simulink model "rtlsdr_am_fdm_demod"  (R2014b)
settings: Solver=ode45  StartTime=0.0  StopTime=60  RelTol=1e-3
PreLoadFcn:
  | %%%%%%%%%%%%%%%%%%%%%%%%%%%%%%%%%%%%%%%%%%%%%%%%%%%%%%%%%%%%%%%%%%%%%%%%%%%
  | % check to see if Simulink library folder is missing from the MATLAB path %
  | %%%%%%%%%%%%%%%%%%%%%%%%%%%%%%%%%%%%%%%%%%%%%%%%%%%%%%%%%%%%%%%%%%%%%%%%%%%
  | if isempty(strfind(path, 'rtlsdr_book_library'))
  | 
  |     % create error window
  |     fig_error = figure(...
  |         'Name', 'Error: RTL-SDR Book Library',...
  |         'Toolbar','none',...
  |         'MenuBar','none',...
  |         'NumberTitle','off',...
  |         'Resize','off',...
  |         'WindowStyle','modal');
  |     fig_error.Position(3) = 600;
  |     fig_error.Position(4) = 150;
  |     fig_axes = axes(...
  |         'Parent',fig_error,...
  |         'Position',[0,0,1,1],...
  |         'visible','off');
  |     % error message
  |     t_title = text(.05,.8,...
  |         'MISSING DIRECTORIES',...
  |         'FontSize',11.5);
  |     t_body = text(.075,.6,...
  |         [{'Simulink cannot find the  \it{<root>}\rm / \it{rtlsdr\_book\_library}\rm  folder in the \it{MATLAB Path}\rm.'},...
  |         {'Please set the MATLAB path following the instructions given in Exercise 2.4.'}],...
  |         'FontSize',10.5);
  |     % buttons
  |     btn_path = uicontrol(...
  |         'Parent',fig_error,...
  |         'String','Set Path Now',...
  |         'FontSize',10,...
  |         'Callback', 'pathtool; close(fig_error);',...
  |         'Position', [fig_error.Position(3)/2-210, 30, 200, 30]);
  |     btn_abort = uicontrol(...
  |         'Parent',fig_error,...
  |         'String','No thanks',...
  |         'FontSize',10,...
  |         'Callback', 'close(fig_error); abort=1;',...
  |         'Position', [fig_error.Position(3)/2+10, 30, 200, 30]);
  | 
  |     % pause to allow user to interact with error box
  |     uiwait(fig_error);
  | 
  |     % abort simulation
  |     try
  |         if abort==1
  |             set_param(gcs, 'SimulationCommand', 'stop');
  |         end
  |     end
  | 
  |     % if user has set path, allow diagram to be updated
  |     if ~exist('abort','var')
  |         % create error window
  |         fig_update = figure(...
  |             'Name', 'Update Diagram',...
  |             'Toolbar','none',...
  |             'MenuBar','none',...
  |             'NumberTitle','off',...
  |             'Resize','off');
  |         fig_update.Position(3) = 400;
  |         fig_update.Position(4) = 120;
  |         fig_axes = axes(...
  |             'Parent',fig_update,...
  |             'Position',[0,0,1,1],...
  |             'visible','off');
  |         % instruction message
  |         t_body = text(.075,.7,...
  |             'Once you have set the path, update the block diagram',...
  |             'FontSize',10.5);
  |         % button
  |         btn_update = uicontrol(...
  |             'Parent',fig_update,...
  |             'String','Update Block Diagram',...
  |             'FontSize',10,...
  |             'Callback', 'set_param(gcs,''SimulationCommand'',''update''); close(gcf)',...
  |             'Position', [fig_update.Position(3)/2-100, 30, 200, 30]);
  |     end
  | 
  |     % clear error components
  |     clear('fig_error','fig_update','fig_axes','t_title','t_body','btn_path','btn_abort','btn_update','abort');
  | 
  | end
  | %%%%%%%%%%%%%%%%%%%%%%%%%%%%%%%%%%%%%%%%%%%%%%%%%%%%%%%%%%%%%%%%%%%%%%%%%%%
undefined symbols (not defined in the file or in its folder): dfilt, fdesignblkfcn, gcbh, startfcn_spectrum_analyzer, startfcn_time_scope
libraries: dsparch4 x4, rtlsdr_book_library x2, dspmlti4 x1, sdrrlib x1, dspsnks4 x1
CloseFcn:
  | closefcn_model;
Description:
  | Software, Simulation Examples and Design Exercises Licence Agreement
  | 
  | This license agreement refers to the simulation examples, design exercises and files,
  | and associated software MATLAB and Simulink resources that accompany the book:
  | 
  |      Title: Software Defined Radio using MATLAB & Simulink and the RTL-SDR
  |      Published by Strathclyde Academic Media, 2015
  |      Authored by Robert W. Stewart, Kenneth W. Barlee, Dale S.W. Atkinson,
  |      and Louise H. Crockett
  | 
  | and made available as a download from, www.desktopSDR.com or variously acquired
  | by other means such as via USB storage, cloud storage, disk or any other electronic
  | or optical or magnetic storage mechanism. These files and associated software may
  | be used subject to the terms of agreement of the conditions below:
  | 
  |     Copyright © 2015 Robert W. Stewart, Kenneth W. Barlee, Dale S.W. Atkinson,
  |     and Louise H. Crockett
  |     All rights reserved.
  | 
  | Redistribution and use in source and binary forms, with or without modification, are
  | permitted provided that the following conditions are met:
  | 
  |    1.  Redistributions of source code must retain the above copyright notice, this list of
  |         conditions and the following disclaimer.
  | 
  |    2.  Redistributions in binary form must reproduce the above copyright notice, this
  |         list of conditions and the following disclaimer in the documentation and/or other
  |         materials provided with the distribution.
  | 
  |    3.  Neither the name of the copyright holder nor the names of its contributors may
  |         be used to endorse or promote products derived from this software without
  |         specific prior written permission.
  | 
  |    4.  In all cases, the software is, and all modifications and derivatives of the
  |         software shall be, licensed to you solely for use in conjunction with The
  |         MathWorks, Inc. products and service offerings.
  | 
  | THIS SOFTWARE IS PROVIDED BY THE COPYRIGHT HOLDERS AND CONTRIBUTORS
  | "AS IS" AND ANY EXPRESS OR IMPLIED WARRANTIES, INCLUDING, BUT NOT LIMITED
  | TO, THE IMPLIED WARRANTIES OF MERCHANTABILITY AND FITNESS FOR A
  | PARTICULAR PURPOSE ARE DISCLAIMED. IN NO EVENT SHALL THE COPYRIGHT
  | HOLDER OR CONTRIBUTORS BE LIABLE FOR ANY DIRECT, INDIRECT, INCIDENTAL,
  | SPECIAL, EXEMPLARY, OR CONSEQUENTIAL DAMAGES (INCLUDING, BUT NOT
  | LIMITED TO, PROCUREMENT OF SUBSTITUTE GOODS OR SERVICES; LOSS OF USE,
  | DATA, OR PROFITS; OR BUSINESS INTERRUPTION) HOWEVER CAUSED AND ON ANY
  | THEORY OF LIABILITY, WHETHER IN CONTRACT, STRICT LIABILITY, OR TORT
  | (INCLUDING NEGLIGENCE OR OTHERWISE) ARISING IN ANY WAY OUT OF THE USE
  | OF THIS SOFTWARE, EVEN IF ADVISED OF THE POSSIBILITY OF SUCH DAMAGE.
  | 
  | 
  | Audio Tracks used in Simulations Examples and Design Exercises
  | 
  | The music and vocal files used within the Examples files and software within the book
  | were variously written, arranged, performed, recorded and produced by Garrey Rice,
  | Adam Struth, Jamie Struth, Iain Thistlethwaite and also Marshall Craigmyle who
  | collectively, and individually where appropriate, assert and retain all of their copyright,
  | performance and artistic rights. Permission to use and reproduce this music is
  | granted for all purposes associated with MATLAB and Simulink software and the
  | simulation examples and design exercises files that accompany this book. Requests to
  | use the music for any other purpose should be directed to: info@desktopSDR.com.
  | For information on music track names, full credits, and links to the musicians please
  | refer to www.desktopSDR.com/more/audio.
settings Model: Creator=desktopSDR Team  LastModifiedBy=desktopSDR Team
settings DataIOCC: LimitDataPoints=off  SaveOutput=off  SignalLogging=off  SaveTime=off

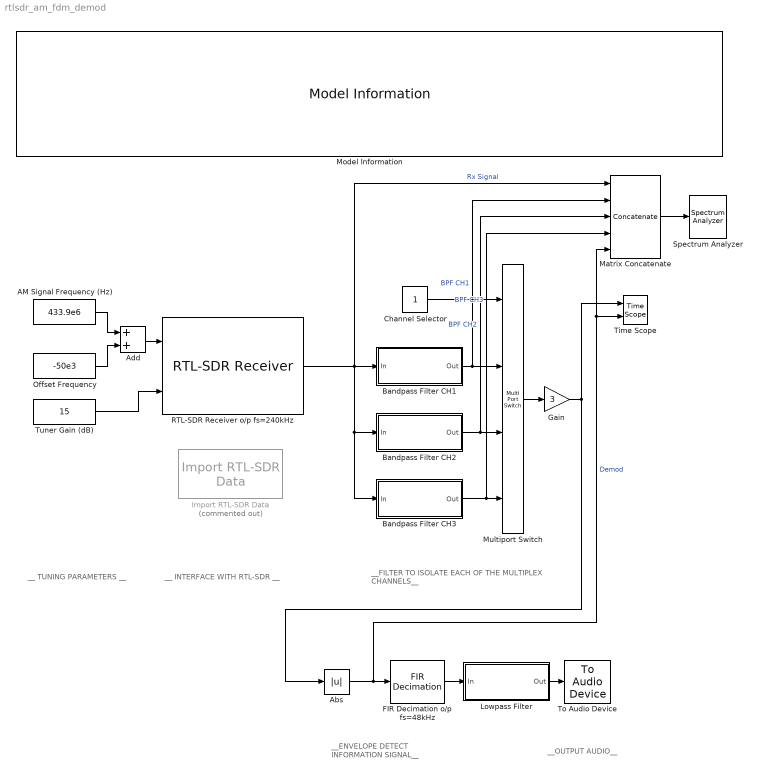
== system rtlsdr_am_fdm_demod ==
  note: __ TUNING PARAMETERS __
  note: __ INTERFACE WITH RTL-SDR __
  note: __FILTER TO ISOLATE EACH
      | OF THE MULTIPLEX CHANNELS__
  note: __OUTPUT AUDIO__
  note: __ENVELOPE DETECT
      | INFORMATION SIGNAL__
  AM Signal Frequency (Hz) : Constant  Value=433.9e6
  Abs : Abs
  Add : Sum
  Bandpass Filter CH1 : Subsystem  DialogController=fdesignblkfcn  InitFcn=fdesignblkfcn(gcbh, {'InitFcn'});  mask(Bandpass Filter){}
      mask help: Design a bandpass filter
      settings: CopyFcn=fdesignblkfcn(gcbh, {'CopyFcn'});
      mask Help: helpview(mapfilelocation('dsp'), 'dspbandpassfilter');
      mask Display: disp('Bandpass');
  Bandpass Filter CH2 : Subsystem  DialogController=fdesignblkfcn  InitFcn=fdesignblkfcn(gcbh, {'InitFcn'});  mask(Bandpass Filter){}
      mask help: Design a bandpass filter
      settings: CopyFcn=fdesignblkfcn(gcbh, {'CopyFcn'});
      mask Help: helpview(mapfilelocation('dsp'), 'dspbandpassfilter');
      mask Display: disp('Bandpass');
  Bandpass Filter CH3 : Subsystem  DialogController=fdesignblkfcn  InitFcn=fdesignblkfcn(gcbh, {'InitFcn'});  mask(Bandpass Filter){}
      mask help: Design a bandpass filter
      settings: CopyFcn=fdesignblkfcn(gcbh, {'CopyFcn'});
      mask Help: helpview(mapfilelocation('dsp'), 'dspbandpassfilter');
      mask Display: disp('Bandpass');
  Channel Selector : Constant
  FIR Decimation o/p fs=48kHz : dspmlti4/FIR Decimation  h=firpm(100, [0 15e3 20e3 (240e3/2)]/(240e3/2), [1 1 0 0], [1 1], 20)  D=5  filtStruct=Direct form  framing=Allow multirate processing  inputOffset=0  outputBufInitCond=0  InputProcessing=Columns as channels (frame based)  firstCoeffDataTypeStr=Inherit: Same word length as input  firstCoeffLastDataTypeStr=Inherit: Same word length as input  firstCoeffMin=[]  firstCoeffMax=[]  outputDataTypeStr=Inherit: Same as accumulator  outputLastDataTypeStr=Inherit: Same as accumulator  outputMin=[]  outputMax=[]  roundingMode=Floor  overflowMode=off  FilterSource=Specify via dialog  FilterObject=Hm_firdecim
      settings: allowOverrides=off
  Gain : Gain  Gain=3
  Import RTL-SDR Data : rtlsdr_book_library/Additional Tools/Import RTL-SDR Data  Commented=on  filename=rec_data/am_fdm.mat  frm_size=4096  data_type=single
  Lowpass Filter : Subsystem  DialogController=fdesignblkfcn  InitFcn=fdesignblkfcn(gcbh, {'InitFcn'});  mask(Lowpass Filter){}
      mask help: Design a lowpass filter
      settings: CopyFcn=fdesignblkfcn(gcbh, {'CopyFcn'});
      mask Help: helpview(mapfilelocation('dsp'), 'dsplowpassfilter');
      mask Display: disp('Lowpass')
  Matrix Concatenate : Concatenate  NumInputs=5  Mode=Multidimensional array  ConcatenateDimension=2
  Model Information : rtlsdr_book_library/Additional Tools/Model Information/Model Information
  Multiport Switch : MultiPortSwitch
  Offset Frequency : Constant  Value=-50e3
  RTL-SDR Receiver o/p fs=240kHz : sdrrlib/RTL-SDR Receiver  SourceLibraryInfo="This block requires <a href=\"http://www.mathworks.com/hardware-support/rtl-sdr.html\">Communications System Toolbox Support Package for RTL-SDR Radio</a>"  sobjType=sdrr.internal.SDRRTLReceiverSL  IPAddress=0  dataUDPPort=-1  ctrlUDPPort=-1  subDeviceList=nosubdev  sdrBlockType=SDRBlockTypeSLT.SDRRxBlock  requester=UNUSED_BY_SFCN  sdrExecutionMode=SDRExecutionModeSLT.ExecModeHW  LostSamplesOutputPort=off  OutputDataType=single  FrameLength=4096  EnableBurstMode=off  NumFramesInBurst=20  BypassUserLogic=off  DecimatorSelect=DDC decimator  SourceSelect=RF data  SineAmplitude=16000  EnableInternalClock=off  BypassIQBalance=off  CenterFrequency=433.9e6-100e3  IFBandwidth=40e6  ADCRateSource=Dialog  ADCRate=240e3  CenterFrequencySource=Input port  GainSource=Input port  IntermediateFrequency=0  Gain=40  DecimationFactorSource=Dialog  DecimationFactor=512  RFFrequencyIsTunable=logical(1)  SampleTime=(4096)/(240e3)  IFBandwidthSource=Dialog  SineFrequency=30000  BypassDCBlockingFilter=off  IntermediateFrequencySource=Dialog  IQBalanceCoefficients=64  SkipAllHardwareResetAndInitialization=off  EnableIQCalibrationTable=on  CacheIQCalibrationTable=off  EnableOffsetTuning=off  EnableRTLAGC=off  EnableTestMode=off  EnableTunerAGC=off  FrequencyCorrectionSource=Dialog  FrequencyCorrection=0  NumMLBuffers=128  NumUSBBuffers=16  LatencyOutputPort=off  RTLCrystalFrequency=28800000  TunerCrystalFrequency=28800000
  Spectrum Analyzer : SpectrumAnalyzer  StartFcn=startfcn_spectrum_analyzer;
  Time Scope : TimeScope  StartFcn=startfcn_time_scope;  DefaultConfigurationName=spbscopes.TimeScopeBlockCfg  NumInputPorts=2
  To Audio Device : dspsnks4/To Audio Device  deviceName=Default  inheritSampleRate=on  sampleRate=44100  deviceDatatype=Determine from input data type  autoBufferSize=on  bufferSize=4096  queueDuration=1.0  defaultOutputChannelMapping=on  outputChannelMapping=1  outputNumUnderrunSamples=off
  Tuner Gain (dB) : Constant  Value=15
  wires:
  AM Signal Frequency (Hz)/1 -> Add/1
  Offset Frequency/1 -> Add/2
  Matrix Concatenate/1 -> Spectrum Analyzer/1
  Add/1 -> RTL-SDR Receiver o/p fs=240kHz/1
  Tuner Gain (dB)/1 -> RTL-SDR Receiver o/p fs=240kHz/2
  Lowpass Filter/1(Out) -> To Audio Device/1
  Channel Selector/1 -> Multiport Switch/1
  Bandpass Filter CH3/1(Out) -> Matrix Concatenate/4, Multiport Switch/4  "BPF CH3"
  Bandpass Filter CH2/1(Out) -> Matrix Concatenate/3, Multiport Switch/3  "BPF CH2"
  FIR Decimation o/p fs=48kHz/1 -> Lowpass Filter/1(In)
  Bandpass Filter CH1/1(Out) -> Matrix Concatenate/2, Multiport Switch/2  "BPF CH1"
  Multiport Switch/1 -> Gain/1
  Abs/1 -> Time Scope/2, Matrix Concatenate/5, FIR Decimation o/p fs=48kHz/1  "Demod"
  Gain/1 -> Time Scope/1, Abs/1
  RTL-SDR Receiver o/p fs=240kHz/1 -> Bandpass Filter CH3/1(In), Bandpass Filter CH2/1(In), Bandpass Filter CH1/1(In), Matrix Concatenate/1  "Rx Signal"

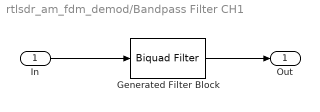
== system rtlsdr_am_fdm_demod/Bandpass Filter CH1 ==
  In : Inport
  Generated Filter Block : dsparch4/Biquad Filter  Tag=BlockMethodSubSystem  IIRFiltStruct=Direct form II  CoeffSource=Specify via dialog  BiQuadCoeffs=[0.48710578309185842 0.020274699864626225 0.47606726400774318 1 -0.3200568934772296 0.9510875417757314;0.61694390478008665 -0.57271773922302893 0.60189559689807448 1 -0.68371663134321814 0.94964854256260212;0.84000114524790004 0.45824504577674063 0.021305946041866301 1 -0.48832315180999453 0.90165549195060035;0.0064548478739541466 0.011389175960501097 0.0049921122031908582 1 -0.72821163596699334 0.034855521810121665;0.77833495194845737 -0.20151009399259803 0.77832234721342286 1 -0.28213942704351702 0.99443660184789129;2 -1.5345249628396347 1.9997202303570027 1 -0.74285445349198365 0.99437926899504725;0.68303493454046227 0.074580654630850063 0.062904140898226851 1 -0.38577358709267945 0.9184389811629543;0.038054397531435698 -0.029838005454256376 0.0052742626653348402 1 -0.60016342729911176 0.91586675515872462;0.81687912100239568 -0.19207817940590149 0.81368134800883141 1 -0.29088293607338106 0.97858989499573013;2 -1.5735978982408823 1.9913568136029411 1 -0.7264857258290689 0.97824331105542206]  a0Flag=Warning  IC=0  ICnum=0  ICden=0  InputProcessing=Columns as channels (frame based)  denAccumFracLength=30  denProdOutputFracLength=30  secondMemoryFracLength=15  roundingMode=Floor  overflowMode=off  ScaleValues=[0.048249460042969664;1;1;1;1;1;1;1;1;1;10.550556890003632]  optimizeScaleValues=off  ScaleValueMode=Specify via input port (g)  scaleValueFracLength=14  FilterSource=Specify via dialog  dfiltObjectName=dfilt.df2tsos([1 0.3 0.4],[1 0.1 0.2])
  Out : Outport
  wires:
  Generated Filter Block/1 -> Out/1
  In/1 -> Generated Filter Block/1

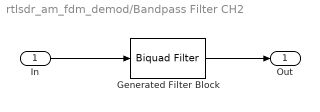
== system rtlsdr_am_fdm_demod/Bandpass Filter CH2 ==
  In : Inport
  Generated Filter Block : dsparch4/Biquad Filter  Tag=BlockMethodSubSystem  IIRFiltStruct=Direct form II  CoeffSource=Specify via dialog  BiQuadCoeffs=[0.67338527760443312 -0.26671696059651728 0.6083593445883243 1 -0.19930278069396612 0.95848462181243144;0.5841637340870659 0.29230149777999481 0.56667307615551432 1 0.19906120642328817 0.9582828801664226;0.149036042446199 0.016946608863773197 0.010962149262872629 1 -0.052041795111932465 0.90786508164551083;0.020481807136560625 0.0032274650327607547 0.00012161868746611722 1 0.051117066171290415 0.9077685137822048;0.88089444047624554 -0.23157465446878642 0.88081993658726632 1 -0.23868838376901563 0.99490529520038307;2 0.52571694552187798 1.9997830967396211 1 0.23871035705725224 0.9948917802055679;0.75363304099796768 -0.50601088924497151 0.63927957482421738 1 -0.14123666236621696 0.929598737259827;0.057396929567661487 0.037309121966942291 0.051540971083893876 1 0.14053864118672826 0.92931947808271609;0.89113560972214434 -0.25188520382892204 0.89037379535859118 1 -0.22797195313135205 0.98116025020292619;2 0.56543358427809076 1.9989110580547198 1 0.22796205762099908 0.98109487138402474]  a0Flag=Warning  IC=0  ICnum=0  ICden=0  InputProcessing=Columns as channels (frame based)  denAccumFracLength=30  denProdOutputFracLength=30  secondMemoryFracLength=15  roundingMode=Floor  overflowMode=off  ScaleValues=[0.041299783151138178;1;1;1;1;1;1;1;1;1;10.556598798294175]  optimizeScaleValues=off  ScaleValueMode=Specify via input port (g)  scaleValueFracLength=14  FilterSource=Specify via dialog  dfiltObjectName=dfilt.df2tsos([1 0.3 0.4],[1 0.1 0.2])
  Out : Outport
  wires:
  Generated Filter Block/1 -> Out/1
  In/1 -> Generated Filter Block/1

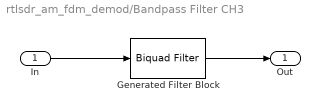
== system rtlsdr_am_fdm_demod/Bandpass Filter CH3 ==
  In : Inport
  Generated Filter Block : dsparch4/Biquad Filter  Tag=BlockMethodSubSystem  IIRFiltStruct=Direct form II  CoeffSource=Specify via dialog  BiQuadCoeffs=[0.60849794827942949 -0.39367779312989598 0.60510522232424568 1 -0.80225454616844827 0.94803791480656774;1.0827491135228735 -1.4017183159916566 1.0805570736721235 1 -1.1330291323642383 0.94553328874405862;-0.28844190743740877 -0.36640640350330222 -0.1161247491557328 1 -0.92719616379501202 0.87407382671627254;0.0051149879255016342 0.0084662498713601719 0.0035008355536301078 1 -0.41129230893568486 0.41217232074731847;0.87875947987193626 -0.67084490391661322 0.87832130941815556 1 -0.78328718222404869 0.99448369227738287;1.6407858750865425 -2 1.6404606425531527 1 -1.1968053935527578 0.99438971688497091;0.95363887304809736 -0.28707398288206454 0.11651775049576317 1 -0.8461554451210308 0.90205598979649637;0.026450365759947799 0.0097397859288686859 0.00089653680768698302 1 -1.0414658285428771 0.89903207911897964;0.76281842819729895 -0.56804251861329702 0.76239803937086215 1 -0.78624791416512241 0.97854881912371261;1.6201527105224738 -2 1.6195618818344955 1 -1.178676630833333 0.97790653821453]  a0Flag=Warning  IC=0  ICnum=0  ICden=0  InputProcessing=Columns as channels (frame based)  denAccumFracLength=30  denProdOutputFracLength=30  secondMemoryFracLength=15  roundingMode=Floor  overflowMode=off  ScaleValues=[0.04734822056392915;1;1;1;1;1;1;1;1;1;16.324610519758114]  optimizeScaleValues=off  ScaleValueMode=Specify via input port (g)  scaleValueFracLength=14  FilterSource=Specify via dialog  dfiltObjectName=dfilt.df2tsos([1 0.3 0.4],[1 0.1 0.2])
  Out : Outport
  wires:
  In/1 -> Generated Filter Block/1
  Generated Filter Block/1 -> Out/1

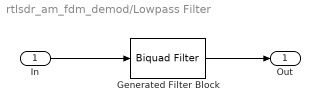
== system rtlsdr_am_fdm_demod/Lowpass Filter ==
  In : Inport
  Generated Filter Block : dsparch4/Biquad Filter  Tag=BlockMethodSubSystem  IIRFiltStruct=Direct form II  CoeffSource=Specify via dialog  BiQuadCoeffs=[0.02505658453151734 0.050113169063034681 0.02505658453151734 1 -1.6618358052504689 0.92327518660477159;0.037716014607021689 0.075432029214043378 0.037716014607021689 1 -1.5666197180702381 0.81307974054400167;0.048494542600695072 0.096989085201390143 0.048494542600695072 1 -1.483833787366122 0.71726995848240305;0.057562689362794101 0.1151253787255882 0.057562689362794101 1 -1.4124095756411101 0.63460931673938947;0.065066669960849324 0.13013333992169865 0.065066669960849324 1 -1.3513355886493104 0.5639271931762575;0.071126049882347511 0.14225209976469502 0.071126049882347511 1 -1.2996951874675289 0.50416274358054824;0.075826965263644491 0.15165393052728898 0.075826965263644491 1 -1.2566848480829704 0.45438603384519421;0.079207708097762716 0.15841541619552543 0.079207708097762716 1 -1.2216205877683222 0.41380547733850032;0.081213644661423695 0.16242728932284739 0.081213644661423695 1 -1.1939377721788489 0.38176761165383055;0.08148106483340975 0.1629621296668195 0.08148106483340975 1 -1.1731876770814522 0.35775311943117882;0.076637308661870573 0.15327461732374115 0.076637308661870573 1 -1.1590329311748637 0.34137155424355531;0.047546496662289287 0.095092993324578573 0.047546496662289287 1 -1.1512431451247189 0.3323562819935113;0.04540058431321875 0.090801168626437501 0.04540058431321875 1 -1.1496915016555413 0.3305605345596806;0.045831247000341468 0.091662494000682937 0.045831247000341468 1 -1.1543527405881076 0.3359550778409825;0.046516257123944797 0.093032514247889594 0.046516257123944797 1 -1.1653027462029997 0.34862773420436555;0.047466760014933662 0.094933520029867324 0.047466760014933662 1 -1.1827197756415799 0.36878480413735909;0.048698191344618065 0.09739638268923613 0.048698191344618065 1 -1.2068872094697505 0.39675424952948513;0.050230457593599342 0.10046091518719868 0.050230457593599342 1 -1.2381975142107695 0.43299027958924174;0.052088101393404251 0.1041762027868085 0.052088101393404251 1 -1.2771568309371673 0.47807866131156473;0.054300385989436643 0.10860077197887329 0.054300385989436643 1 -1.3243891792379572 0.53274158481157419;0.056901193140924844 0.11380238628184969 0.056901193140924844 1 -1.3806386047689676 0.59784014872671409;0.059928568932260555 0.11985713786452111 0.059928568932260555 1 -1.4467665832625731 0.6743713558262725;0.063423665332839996 0.12684733066567999 0.063423665332839996 1 -1.5237404723519465 0.76345474808098879;0.023993836801624483 0.047987673603248966 0.023993836801624483 1 -1.612606599730263 0.86630126106162297;0.014199710532717848 0.028399421065435696 0.014199710532717848 1 -1.7144385404499303 0.98415336424243371;0.028453803345255303 0.056907606690510606 0.028453803345255303 1 -1.6368075882726612 0.89430953998294882;0.04083171761385794 0.08166343522771588 0.04083171761385794 1 -1.5448001049050344 0.78782747407497666;0.051459392354549008 0.10291878470909802 0.051459392354549008 1 -1.4649534370622368 0.69541935859814075;0.060531990296125222 0.12106398059225044 0.060531990296125222 1 -1.3962083671487442 0.61585934024476119;0.06815377125244737 0.13630754250489474 0.06815377125244737 1 -1.3375744913620335 0.54800120526008977;0.074455848419753085 0.14891169683950617 0.074455848419753085 1 -1.2881623105057174 0.49081551877004753;0.079552479596548167 0.15910495919309633 0.079552479596548167 1 -1.2471979145071224 0.44340661946156557;0.083510197687583193 0.16702039537516639 0.083510197687583193 1 -1.2140273488611264 0.40501767295371627;0.086395360489223874 0.17279072097844775 0.086395360489223874 1 -1.1881153515668013 0.37502921002970635;0.08825814050628647 0.17651628101257294 0.08825814050628647 1 -1.1690414739763555 0.35295463721924042;0.072653340568011524 0.14530668113602305 0.072653340568011524 1 -1.1564954726095342 0.33843490365490059;0.10631278825624907 0.21262557651249814 0.10631278825624907 1 -1.150273121708774 0.33123365486006179;0.09066349956390464 0.09066349956390464 0 1 -0.57474884697500372 0;0.045700079748393248 0.091400159496786496 0.045700079748393248 1 -1.1526025576110279 ...(+1167 chars)Flag=Warning  IC=0  ICnum=0  ICden=0  InputProcessing=Columns as channels (frame based)  denAccumFracLength=30  denProdOutputFracLength=30  secondMemoryFracLength=15  roundingMode=Floor  overflowMode=off  ScaleValues=[0.038531123333914737;1;1;1;1;1;1;1;1;1;1;1;1;1;1;1;1;1;1;1;1;1;1;1;1;1;1;1;1;1;1;1;1;1;1;1;1;1;1;1;1;1;1;1;1;1;1;1;1;1;1]  optimizeScaleValues=off  ScaleValueMode=Specify via input port (g)  scaleValueFracLength=14  FilterSource=Specify via dialog  dfiltObjectName=dfilt.df2tsos([1 0.3 0.4],[1 0.1 0.2])
  Out : Outport
  wires:
  Generated Filter Block/1 -> Out/1
  In/1 -> Generated Filter Block/1
